simulink model "HANcoder_E407_TTA_Controller_v3"  (R2018b)
settings: Solver=FixedStepDiscrete  StartTime=0.0  StopTime=1  FixedStep=0.01  RelTol=1e-3
PreLoadFcn:
  | librarySetup
  | eval([bdroot,'_startup']) %Calling [modelName]_startup.m
values from neighbouring files (symbols this model uses):
  basic_cycle_duration_bc0 = TM_Reset_Board   + COMP_duration    (= 212)    [HANcoder_E407_TTA_Controller_v3_5_startup.m]    (also in HANcoder_E407_TTA_Controller_v4_6_startup.m; HANcoder_E407_TTA_Controller_v4_7_startup.m; HANcoder_E407_TTA_Controller_v4_startup.m)
  basic_cycle_duration_bc1 = TM_Reset_Var_bc1 + COMP_duration    (= 288)    [HANcoder_E407_TTA_Controller_v3_5_startup.m]    (also in HANcoder_E407_TTA_Controller_v4_6_startup.m = 332; HANcoder_E407_TTA_Controller_v4_7_startup.m = 372; HANcoder_E407_TTA_Controller_v4_startup.m = 332)
  comm_delay_estimation1 = round(comm_delay_measured1*hardware_granularity/frequency_IRQ)    [HANcoder_E407_TTA_Controller_v3_5_startup.m]    (also in HANcoder_E407_TTA_Controller_v4_6_startup.m; HANcoder_E407_TTA_Controller_v4_7_startup.m; HANcoder_E407_TTA_Controller_v4_startup.m)
  comm_delay_estimation2 = round(comm_delay_measured2*hardware_granularity/frequency_IRQ)    [HANcoder_E407_TTA_Controller_v3_5_startup.m]    (also in HANcoder_E407_TTA_Controller_v4_6_startup.m; HANcoder_E407_TTA_Controller_v4_7_startup.m; HANcoder_E407_TTA_Controller_v4_startup.m)
  COMM_Period = 40    [HANcoder_E407_TTA_Controller_v3_5_startup.m]    (also in HANcoder_E407_TTA_Controller_v4_6_startup.m; HANcoder_E407_TTA_Controller_v4_7_startup.m; HANcoder_E407_TTA_Controller_v4_startup.m)
  COMM_Phase1 = Simulink.Parameter    [HANcoder_E407_TTA_Controller_v3_5_startup.m]    (also in HANcoder_E407_TTA_Controller_v4_6_startup.m; HANcoder_E407_TTA_Controller_v4_7_startup.m; HANcoder_E407_TTA_Controller_v4_startup.m)
  COMM_Phase2 = Simulink.Parameter    [HANcoder_E407_TTA_Controller_v3_5_startup.m]    (also in HANcoder_E407_TTA_Controller_v4_6_startup.m; HANcoder_E407_TTA_Controller_v4_7_startup.m; HANcoder_E407_TTA_Controller_v4_startup.m)
  COMM_Phase_init1 = Simulink.Parameter    [HANcoder_E407_TTA_Controller_v3_5_startup.m]    (also in HANcoder_E407_TTA_Controller_v4_6_startup.m; HANcoder_E407_TTA_Controller_v4_7_startup.m; HANcoder_E407_TTA_Controller_v4_startup.m)
  COMM_Phase_init2 = Simulink.Parameter    [HANcoder_E407_TTA_Controller_v3_5_startup.m]    (also in HANcoder_E407_TTA_Controller_v4_6_startup.m; HANcoder_E407_TTA_Controller_v4_7_startup.m; HANcoder_E407_TTA_Controller_v4_startup.m)
  COMP_duration = 4    [HANcoder_E407_TTA_Controller_v3_5_startup.m]    (also in HANcoder_E407_TTA_Controller_v4_6_startup.m; HANcoder_E407_TTA_Controller_v4_7_startup.m; HANcoder_E407_TTA_Controller_v4_startup.m)
  Controller1_Board = 1    [HANcoder_E407_TTA_Controller_v3_5_startup.m]    (also in HANcoder_E407_TTA_Controller_v4_6_startup.m; HANcoder_E407_TTA_Controller_v4_7_startup.m; HANcoder_E407_TTA_Controller_v4_startup.m)
  Controller2_Board = 2    [HANcoder_E407_TTA_Controller_v3_5_startup.m]    (also in HANcoder_E407_TTA_Controller_v4_6_startup.m; HANcoder_E407_TTA_Controller_v4_7_startup.m; HANcoder_E407_TTA_Controller_v4_startup.m)
  Controller3_Board = 3    [HANcoder_E407_TTA_Controller_v3_5_startup.m]    (also in HANcoder_E407_TTA_Controller_v4_6_startup.m; HANcoder_E407_TTA_Controller_v4_7_startup.m; HANcoder_E407_TTA_Controller_v4_startup.m)
  delta_a_set = Simulink.Parameter    [HANcoder_E407_TTA_Controller_v3_5_startup.m]    (also in HANcoder_E407_TTA_Controller_v4_6_startup.m; HANcoder_E407_TTA_Controller_v4_7_startup.m; HANcoder_E407_TTA_Controller_v4_startup.m)
  delta_f_set = Simulink.Parameter    [HANcoder_E407_TTA_Controller_v3_5_startup.m]    (also in HANcoder_E407_TTA_Controller_v4_6_startup.m; HANcoder_E407_TTA_Controller_v4_7_startup.m; HANcoder_E407_TTA_Controller_v4_startup.m)
  delta_max = 1    [HANcoder_E407_TTA_Controller_v3_5_startup.m]    (also in HANcoder_E407_TTA_Controller_v4_6_startup.m; HANcoder_E407_TTA_Controller_v4_7_startup.m; HANcoder_E407_TTA_Controller_v4_startup.m)
  delta_min = -1    [HANcoder_E407_TTA_Controller_v3_5_startup.m]    (also in HANcoder_E407_TTA_Controller_v4_6_startup.m; HANcoder_E407_TTA_Controller_v4_7_startup.m; HANcoder_E407_TTA_Controller_v4_startup.m)
  delta_precision = 6    [HANcoder_E407_TTA_Controller_v3_5_startup.m]    (also in HANcoder_E407_TTA_Controller_v4_6_startup.m; HANcoder_E407_TTA_Controller_v4_7_startup.m; HANcoder_E407_TTA_Controller_v4_startup.m)
  e_width = 0.1    [HANcoder_E407_TTA_Controller_v3_5_startup.m]    (also in HANcoder_E407_TTA_Controller_v4_6_startup.m; HANcoder_E407_TTA_Controller_v4_7_startup.m; HANcoder_E407_TTA_Controller_v4_startup.m)
  frequency_IRQ = 100    [HANcoder_E407_2xCAN_TEST_startup.m]    (also in HANcoder_E407_TTA_Controller_v3_5_startup.m; HANcoder_E407_TTA_Controller_v4_6_startup.m; HANcoder_E407_TTA_Controller_v4_7_startup.m; HANcoder_E407_TTA_Controller_v4_startup.m)
  HANtuneOverride = Simulink.Parameter    [HANcoder_E407_2xCAN_TEST_startup.m]    (also in HANcoder_E407_TTA_Controller_v3_5_startup.m; HANcoder_E407_TTA_Controller_v4_6_startup.m; HANcoder_E407_TTA_Controller_v4_7_startup.m; HANcoder_E407_TTA_Controller_v4_startup.m)
  hardware_granularity = 1000000    [HANcoder_E407_2xCAN_TEST_startup.m]    (also in HANcoder_E407_TTA_Controller_v3_5_startup.m; HANcoder_E407_TTA_Controller_v4_6_startup.m; HANcoder_E407_TTA_Controller_v4_7_startup.m; HANcoder_E407_TTA_Controller_v4_startup.m)
  I_a = 2.25    [HANcoder_E407_TTA_Controller_v3_5_startup.m]    (also in HANcoder_E407_TTA_Controller_v4_6_startup.m; HANcoder_E407_TTA_Controller_v4_7_startup.m; HANcoder_E407_TTA_Controller_v4_startup.m)
  I_f = 2.25    [HANcoder_E407_TTA_Controller_v3_5_startup.m]    (also in HANcoder_E407_TTA_Controller_v4_6_startup.m; HANcoder_E407_TTA_Controller_v4_7_startup.m; HANcoder_E407_TTA_Controller_v4_startup.m)
  idle_time_init = basic_cycle_duration_bc0 + basic_cycle_duration_bc1    (= 500)    [HANcoder_E407_TTA_Controller_v3_5_startup.m]    (also in HANcoder_E407_TTA_Controller_v4_6_startup.m = 544; HANcoder_E407_TTA_Controller_v4_7_startup.m = 584; HANcoder_E407_TTA_Controller_v4_startup.m = 544)
  Input_Gen_Board = 4    [HANcoder_E407_TTA_Controller_v3_5_startup.m]    (also in HANcoder_E407_TTA_Controller_v4_6_startup.m; HANcoder_E407_TTA_Controller_v4_7_startup.m; HANcoder_E407_TTA_Controller_v4_startup.m)
  LA_Clock_Gr = 1    [HANcoder_E407_TTA_Controller_v3_5_startup.m]    (also in HANcoder_E407_TTA_Controller_v4_6_startup.m; HANcoder_E407_TTA_Controller_v4_7_startup.m; HANcoder_E407_TTA_Controller_v4_startup.m)
  LA_COMM_dly = 1    [HANcoder_E407_TTA_Controller_v3_5_startup.m]    (also in HANcoder_E407_TTA_Controller_v4_6_startup.m; HANcoder_E407_TTA_Controller_v4_7_startup.m; HANcoder_E407_TTA_Controller_v4_startup.m)
  LA_COMM_Err = 1    [HANcoder_E407_TTA_Controller_v3_5_startup.m]    (also in HANcoder_E407_TTA_Controller_v4_6_startup.m; HANcoder_E407_TTA_Controller_v4_7_startup.m; HANcoder_E407_TTA_Controller_v4_startup.m)
  LA_E_Desync = 1    [HANcoder_E407_TTA_Controller_v3_5_startup.m]    (also in HANcoder_E407_TTA_Controller_v4_6_startup.m; HANcoder_E407_TTA_Controller_v4_7_startup.m; HANcoder_E407_TTA_Controller_v4_startup.m)
  LA_MEX_Flag = 1    [HANcoder_E407_TTA_Controller_v3_5_startup.m]    (also in HANcoder_E407_TTA_Controller_v4_6_startup.m; HANcoder_E407_TTA_Controller_v4_7_startup.m; HANcoder_E407_TTA_Controller_v4_startup.m)
  LA_Task_Act = 1    [HANcoder_E407_TTA_Controller_v3_5_startup.m]    (also in HANcoder_E407_TTA_Controller_v4_6_startup.m; HANcoder_E407_TTA_Controller_v4_7_startup.m; HANcoder_E407_TTA_Controller_v4_startup.m)
  m_v = 100.0    (= 100)    [HANcoder_E407_TTA_Controller_v3_5_startup.m]    (also in HANcoder_E407_TTA_Controller_v4_6_startup.m; HANcoder_E407_TTA_Controller_v4_7_startup.m; HANcoder_E407_TTA_Controller_v4_startup.m)
  Master_Role = 1    [HANcoder_E407_TTA_Controller_v3_5_startup.m]    (also in HANcoder_E407_TTA_Controller_v4_6_startup.m; HANcoder_E407_TTA_Controller_v4_7_startup.m; HANcoder_E407_TTA_Controller_v4_startup.m)
  matrix_cycle_duration = basic_cycle_duration_bc0 + basic_cycle_duration_bc1    (= 500)    [HANcoder_E407_TTA_Controller_v3_5_startup.m]    (also in HANcoder_E407_TTA_Controller_v4_6_startup.m = 544; HANcoder_E407_TTA_Controller_v4_7_startup.m = 584; HANcoder_E407_TTA_Controller_v4_startup.m = 544)
  matrix_rows = 2    [HANcoder_E407_TTA_Controller_v3_5_startup.m]    (also in HANcoder_E407_TTA_Controller_v4_6_startup.m; HANcoder_E407_TTA_Controller_v4_7_startup.m; HANcoder_E407_TTA_Controller_v4_startup.m)
  max_desync = 15    [HANcoder_E407_TTA_Controller_v3_5_startup.m]    (also in HANcoder_E407_TTA_Controller_v4_6_startup.m; HANcoder_E407_TTA_Controller_v4_7_startup.m = 30; HANcoder_E407_TTA_Controller_v4_startup.m)
  max_num_msgs_CAN1 = 2^Tx_bit_number-1    (= 7)    [HANcoder_E407_TTA_Controller_v3_5_startup.m]    (also in HANcoder_E407_TTA_Controller_v4_6_startup.m = 15; HANcoder_E407_TTA_Controller_v4_7_startup.m = 15; HANcoder_E407_TTA_Controller_v4_startup.m)
  max_num_msgs_CAN2 = max_num_msgs_CAN1    (= 7)    [HANcoder_E407_TTA_Controller_v3_5_startup.m]    (also in HANcoder_E407_TTA_Controller_v4_6_startup.m = 15; HANcoder_E407_TTA_Controller_v4_7_startup.m = 15; HANcoder_E407_TTA_Controller_v4_startup.m)
  min_desync = (-1)*max_desync    (= -15)    [HANcoder_E407_TTA_Controller_v3_5_startup.m]    (also in HANcoder_E407_TTA_Controller_v4_6_startup.m; HANcoder_E407_TTA_Controller_v4_7_startup.m = -30; HANcoder_E407_TTA_Controller_v4_startup.m)
  OutControl1_ID = 23    [HANcoder_E407_TTA_Controller_v3_5_startup.m]    (also in HANcoder_E407_TTA_Controller_v4_6_startup.m; HANcoder_E407_TTA_Controller_v4_7_startup.m; HANcoder_E407_TTA_Controller_v4_startup.m)
  OutControl2_ID = 24    [HANcoder_E407_TTA_Controller_v3_5_startup.m]    (also in HANcoder_E407_TTA_Controller_v4_6_startup.m; HANcoder_E407_TTA_Controller_v4_7_startup.m; HANcoder_E407_TTA_Controller_v4_startup.m)
  OutEmulator_ID = 25    [HANcoder_E407_TTA_Controller_v3_5_startup.m]    (also in HANcoder_E407_TTA_Controller_v4_6_startup.m = 26; HANcoder_E407_TTA_Controller_v4_7_startup.m = 26; HANcoder_E407_TTA_Controller_v4_startup.m)
  R_al = 0.10    (= 0.1)    [HANcoder_E407_TTA_Controller_v3_5_startup.m]    (also in HANcoder_E407_TTA_Controller_v4_6_startup.m; HANcoder_E407_TTA_Controller_v4_7_startup.m; HANcoder_E407_TTA_Controller_v4_startup.m)
  R_ar = 0.10    (= 0.1)    [HANcoder_E407_TTA_Controller_v3_5_startup.m]    (also in HANcoder_E407_TTA_Controller_v4_6_startup.m; HANcoder_E407_TTA_Controller_v4_7_startup.m; HANcoder_E407_TTA_Controller_v4_startup.m)
  R_fl = 0.10    (= 0.1)    [HANcoder_E407_TTA_Controller_v3_5_startup.m]    (also in HANcoder_E407_TTA_Controller_v4_6_startup.m; HANcoder_E407_TTA_Controller_v4_7_startup.m; HANcoder_E407_TTA_Controller_v4_startup.m)
  R_fr = 0.10    (= 0.1)    [HANcoder_E407_TTA_Controller_v3_5_startup.m]    (also in HANcoder_E407_TTA_Controller_v4_6_startup.m; HANcoder_E407_TTA_Controller_v4_7_startup.m; HANcoder_E407_TTA_Controller_v4_startup.m)
  script_run = Simulink.Parameter    [HANcoder_E407_TTA_Controller_v3_5_startup.m]    (also in HANcoder_E407_TTA_Controller_v4_6_startup.m; HANcoder_E407_TTA_Controller_v4_7_startup.m; HANcoder_E407_TTA_Controller_v4_startup.m)
  SensorValues_ID = 22    [HANcoder_E407_TTA_Controller_v3_5_startup.m]    (also in HANcoder_E407_TTA_Controller_v4_6_startup.m; HANcoder_E407_TTA_Controller_v4_7_startup.m; HANcoder_E407_TTA_Controller_v4_startup.m)
  SetValues_ID = 21    [HANcoder_E407_TTA_Controller_v3_5_startup.m]    (also in HANcoder_E407_TTA_Controller_v4_6_startup.m; HANcoder_E407_TTA_Controller_v4_7_startup.m; HANcoder_E407_TTA_Controller_v4_startup.m)
  Slave_Role = 2    [HANcoder_E407_TTA_Controller_v3_5_startup.m]    (also in HANcoder_E407_TTA_Controller_v4_6_startup.m; HANcoder_E407_TTA_Controller_v4_7_startup.m; HANcoder_E407_TTA_Controller_v4_startup.m)
  speed_k_d = Simulink.Parameter    [HANcoder_E407_TTA_Controller_v3_5_startup.m]    (also in HANcoder_E407_TTA_Controller_v4_6_startup.m; HANcoder_E407_TTA_Controller_v4_7_startup.m; HANcoder_E407_TTA_Controller_v4_startup.m)
  speed_k_i = Simulink.Parameter    [HANcoder_E407_TTA_Controller_v3_5_startup.m]    (also in HANcoder_E407_TTA_Controller_v4_6_startup.m; HANcoder_E407_TTA_Controller_v4_7_startup.m; HANcoder_E407_TTA_Controller_v4_startup.m)
  speed_k_p = Simulink.Parameter    [HANcoder_E407_TTA_Controller_v3_5_startup.m]    (also in HANcoder_E407_TTA_Controller_v4_6_startup.m; HANcoder_E407_TTA_Controller_v4_7_startup.m; HANcoder_E407_TTA_Controller_v4_startup.m)
  speed_max = 10    [HANcoder_E407_TTA_Controller_v3_5_startup.m]    (also in HANcoder_E407_TTA_Controller_v4_6_startup.m; HANcoder_E407_TTA_Controller_v4_7_startup.m; HANcoder_E407_TTA_Controller_v4_startup.m)
  speed_min = -10    [HANcoder_E407_TTA_Controller_v3_5_startup.m]    (also in HANcoder_E407_TTA_Controller_v4_6_startup.m; HANcoder_E407_TTA_Controller_v4_7_startup.m; HANcoder_E407_TTA_Controller_v4_startup.m)
  speed_precision = 3    [HANcoder_E407_TTA_Controller_v3_5_startup.m]    (also in HANcoder_E407_TTA_Controller_v4_6_startup.m; HANcoder_E407_TTA_Controller_v4_7_startup.m; HANcoder_E407_TTA_Controller_v4_startup.m)
  Sync_ID = 1    [HANcoder_E407_TTA_Controller_v3_5_startup.m]    (also in HANcoder_E407_TTA_Controller_v4_6_startup.m; HANcoder_E407_TTA_Controller_v4_7_startup.m; HANcoder_E407_TTA_Controller_v4_startup.m)
  tau_max = 5    [HANcoder_E407_TTA_Controller_v3_5_startup.m]    (also in HANcoder_E407_TTA_Controller_v4_6_startup.m; HANcoder_E407_TTA_Controller_v4_7_startup.m; HANcoder_E407_TTA_Controller_v4_startup.m)
  tau_min = -5    [HANcoder_E407_TTA_Controller_v3_5_startup.m]    (also in HANcoder_E407_TTA_Controller_v4_6_startup.m; HANcoder_E407_TTA_Controller_v4_7_startup.m; HANcoder_E407_TTA_Controller_v4_startup.m)
  tau_range = abs(tau_max) + abs(tau_min)    [HANcoder_E407_TTA_Controller_v3_5_startup.m]    (also in HANcoder_E407_TTA_Controller_v4_6_startup.m; HANcoder_E407_TTA_Controller_v4_7_startup.m; HANcoder_E407_TTA_Controller_v4_startup.m)
  theta_max = (speed_max/R_fr)*matrix_cycle_duration*frequency_IRQ/hardware_granularity    (= 5)    [HANcoder_E407_TTA_Controller_v3_5_startup.m]    (also in HANcoder_E407_TTA_Controller_v4_6_startup.m = 5.44; HANcoder_E407_TTA_Controller_v4_7_startup.m = 5.84; HANcoder_E407_TTA_Controller_v4_startup.m = 5.44)
  theta_min = (-1)*theta_max    (= -5)    [HANcoder_E407_TTA_Controller_v3_5_startup.m]    (also in HANcoder_E407_TTA_Controller_v4_6_startup.m = -5.44; HANcoder_E407_TTA_Controller_v4_7_startup.m = -5.84; HANcoder_E407_TTA_Controller_v4_startup.m = -5.44)
  theta_precision = 7-(fix(log2(theta_max))+1)    [HANcoder_E407_TTA_Controller_v3_5_startup.m]    (also in HANcoder_E407_TTA_Controller_v4_6_startup.m; HANcoder_E407_TTA_Controller_v4_7_startup.m; HANcoder_E407_TTA_Controller_v4_startup.m)
  Tl_a = 0.6    [HANcoder_E407_TTA_Controller_v3_5_startup.m]    (also in HANcoder_E407_TTA_Controller_v4_6_startup.m; HANcoder_E407_TTA_Controller_v4_7_startup.m; HANcoder_E407_TTA_Controller_v4_startup.m)
  Tl_f = 0.6    [HANcoder_E407_TTA_Controller_v3_5_startup.m]    (also in HANcoder_E407_TTA_Controller_v4_6_startup.m; HANcoder_E407_TTA_Controller_v4_7_startup.m; HANcoder_E407_TTA_Controller_v4_startup.m)
  TM_Check_Output_Control1 = TM_COMM_Output_Control1 + COMM_duration    (= 188)    [HANcoder_E407_TTA_Controller_v3_5_startup.m]    (also in HANcoder_E407_TTA_Controller_v4_6_startup.m; HANcoder_E407_TTA_Controller_v4_7_startup.m; HANcoder_E407_TTA_Controller_v4_startup.m)
  TM_Check_Output_Control2 = TM_COMM_Output_Control2 + COMM_duration    (= 232)    [HANcoder_E407_TTA_Controller_v3_5_startup.m]    (also in HANcoder_E407_TTA_Controller_v4_6_startup.m; HANcoder_E407_TTA_Controller_v4_7_startup.m; HANcoder_E407_TTA_Controller_v4_startup.m)
  TM_Check_Output_Emulator = TM_COMM_Output_Emulator + COMM_duration    (= 280)    [HANcoder_E407_TTA_Controller_v3_5_startup.m]    (also in HANcoder_E407_TTA_Controller_v4_6_startup.m = 320; HANcoder_E407_TTA_Controller_v4_7_startup.m = 360; HANcoder_E407_TTA_Controller_v4_startup.m = 320)
  TM_Check_Output_Emulator_2 = TM_Check_Output_Emulator + 2    (= 282)    [HANcoder_E407_TTA_Controller_v3_5_startup.m]    (also in HANcoder_E407_TTA_Controller_v4_6_startup.m = 322; HANcoder_E407_TTA_Controller_v4_7_startup.m = 362; HANcoder_E407_TTA_Controller_v4_startup.m = 322)
  TM_Check_Sensor_Values = TM_COMM_Sensor_Values + COMM_duration    (= 132)    [HANcoder_E407_TTA_Controller_v3_5_startup.m]    (also in HANcoder_E407_TTA_Controller_v4_6_startup.m; HANcoder_E407_TTA_Controller_v4_7_startup.m; HANcoder_E407_TTA_Controller_v4_startup.m)
  TM_Check_Sensor_Values_2 = TM_Check_Sensor_Values + 2    (= 134)    [HANcoder_E407_TTA_Controller_v3_5_startup.m]    (also in HANcoder_E407_TTA_Controller_v4_6_startup.m; HANcoder_E407_TTA_Controller_v4_7_startup.m; HANcoder_E407_TTA_Controller_v4_startup.m)
  TM_Check_Set_Values = TM_COMM_Set_Values + COMM_duration    (= 88)    [HANcoder_E407_TTA_Controller_v3_5_startup.m]    (also in HANcoder_E407_TTA_Controller_v4_6_startup.m; HANcoder_E407_TTA_Controller_v4_7_startup.m; HANcoder_E407_TTA_Controller_v4_startup.m)
  TM_Check_Set_Values_2 = TM_Check_Set_Values + 2    (= 90)    [HANcoder_E407_TTA_Controller_v3_5_startup.m]    (also in HANcoder_E407_TTA_Controller_v4_6_startup.m; HANcoder_E407_TTA_Controller_v4_7_startup.m; HANcoder_E407_TTA_Controller_v4_startup.m)
  TM_Check_Sync = TM_COMM_Sync   + COMM_duration    (= 40)    [HANcoder_E407_TTA_Controller_v3_5_startup.m]    (also in HANcoder_E407_TTA_Controller_v4_6_startup.m; HANcoder_E407_TTA_Controller_v4_7_startup.m; HANcoder_E407_TTA_Controller_v4_startup.m)
  TM_Check_TOuts = TM_Count_Vote3 + COMP_duration    (= 196)    [HANcoder_E407_TTA_Controller_v3_5_startup.m]    (also in HANcoder_E407_TTA_Controller_v4_6_startup.m; HANcoder_E407_TTA_Controller_v4_7_startup.m; HANcoder_E407_TTA_Controller_v4_startup.m)
  TM_Check_Vote1 = TM_COMM_Vote1  + COMM_duration    (= 92)    [HANcoder_E407_TTA_Controller_v3_5_startup.m]    (also in HANcoder_E407_TTA_Controller_v4_6_startup.m; HANcoder_E407_TTA_Controller_v4_7_startup.m; HANcoder_E407_TTA_Controller_v4_startup.m)
  TM_Check_Vote2 = TM_COMM_Vote2  + COMM_duration    (= 140)    [HANcoder_E407_TTA_Controller_v3_5_startup.m]    (also in HANcoder_E407_TTA_Controller_v4_6_startup.m; HANcoder_E407_TTA_Controller_v4_7_startup.m; HANcoder_E407_TTA_Controller_v4_startup.m)
  TM_Check_Vote2_2 = TM_Check_Vote2 + 2    (= 142)    [HANcoder_E407_TTA_Controller_v3_5_startup.m]    (also in HANcoder_E407_TTA_Controller_v4_6_startup.m; HANcoder_E407_TTA_Controller_v4_7_startup.m; HANcoder_E407_TTA_Controller_v4_startup.m)
  TM_Check_Vote3 = TM_COMM_Vote3  + COMM_duration    (= 188)    [HANcoder_E407_TTA_Controller_v3_5_startup.m]    (also in HANcoder_E407_TTA_Controller_v4_6_startup.m; HANcoder_E407_TTA_Controller_v4_7_startup.m; HANcoder_E407_TTA_Controller_v4_startup.m)
  TM_COMM_Output_Control1 = TM_Velocity + COMP_duration    (= 148)    [HANcoder_E407_TTA_Controller_v3_5_startup.m]    (also in HANcoder_E407_TTA_Controller_v4_6_startup.m; HANcoder_E407_TTA_Controller_v4_7_startup.m; HANcoder_E407_TTA_Controller_v4_startup.m)
  TM_COMM_Output_Control2 = TM_Check_Output_Control1 + COMP_duration    (= 192)    [HANcoder_E407_TTA_Controller_v3_5_startup.m]    (also in HANcoder_E407_TTA_Controller_v4_6_startup.m; HANcoder_E407_TTA_Controller_v4_7_startup.m; HANcoder_E407_TTA_Controller_v4_startup.m)
  TM_COMM_Output_Emulator = TM_TMR + COMP_duration    (= 240)    [HANcoder_E407_TTA_Controller_v3_5_startup.m]    (also in HANcoder_E407_TTA_Controller_v4_6_startup.m = 280; HANcoder_E407_TTA_Controller_v4_7_startup.m = 320; HANcoder_E407_TTA_Controller_v4_startup.m = 280)
  TM_COMM_Sensor_Values = TM_Check_Set_Values + COMP_duration    (= 92)    [HANcoder_E407_TTA_Controller_v3_5_startup.m]    (also in HANcoder_E407_TTA_Controller_v4_6_startup.m; HANcoder_E407_TTA_Controller_v4_7_startup.m; HANcoder_E407_TTA_Controller_v4_startup.m)
  TM_COMM_Set_Values = TM_Update_LT + COMP_duration    (= 48)    [HANcoder_E407_TTA_Controller_v3_5_startup.m]    (also in HANcoder_E407_TTA_Controller_v4_6_startup.m; HANcoder_E407_TTA_Controller_v4_7_startup.m; HANcoder_E407_TTA_Controller_v4_startup.m)
  TM_COMM_Sync = basic_cycle_start    (= 0)    [HANcoder_E407_TTA_Controller_v3_5_startup.m]    (also in HANcoder_E407_TTA_Controller_v4_6_startup.m; HANcoder_E407_TTA_Controller_v4_7_startup.m; HANcoder_E407_TTA_Controller_v4_startup.m)
  TM_COMM_Vote1 = TM_Vote_Dec    + COMP_duration    (= 52)    [HANcoder_E407_TTA_Controller_v3_5_startup.m]    (also in HANcoder_E407_TTA_Controller_v4_6_startup.m; HANcoder_E407_TTA_Controller_v4_7_startup.m; HANcoder_E407_TTA_Controller_v4_startup.m)
  TM_COMM_Vote2 = TM_Count_Vote1 + COMP_duration    (= 100)    [HANcoder_E407_TTA_Controller_v3_5_startup.m]    (also in HANcoder_E407_TTA_Controller_v4_6_startup.m; HANcoder_E407_TTA_Controller_v4_7_startup.m; HANcoder_E407_TTA_Controller_v4_startup.m)
  TM_COMM_Vote3 = TM_Count_Vote2 + COMP_duration    (= 148)    [HANcoder_E407_TTA_Controller_v3_5_startup.m]    (also in HANcoder_E407_TTA_Controller_v4_6_startup.m; HANcoder_E407_TTA_Controller_v4_7_startup.m; HANcoder_E407_TTA_Controller_v4_startup.m)
  TM_Count_Vote1 = TM_Check_Vote1 + COMP_duration    (= 96)    [HANcoder_E407_TTA_Controller_v3_5_startup.m]    (also in HANcoder_E407_TTA_Controller_v4_6_startup.m; HANcoder_E407_TTA_Controller_v4_7_startup.m; HANcoder_E407_TTA_Controller_v4_startup.m)
  TM_Count_Vote2 = TM_Check_Vote2 + COMP_duration    (= 144)    [HANcoder_E407_TTA_Controller_v3_5_startup.m]    (also in HANcoder_E407_TTA_Controller_v4_6_startup.m; HANcoder_E407_TTA_Controller_v4_7_startup.m; HANcoder_E407_TTA_Controller_v4_startup.m)
  TM_Count_Vote3 = TM_Check_Vote3 + COMP_duration    (= 192)    [HANcoder_E407_TTA_Controller_v3_5_startup.m]    (also in HANcoder_E407_TTA_Controller_v4_6_startup.m; HANcoder_E407_TTA_Controller_v4_7_startup.m; HANcoder_E407_TTA_Controller_v4_startup.m)
  TM_Data_bc0 = TM_COMM_Sync    (= 0)    [HANcoder_E407_TTA_Controller_v3_5_startup.m]    (also in HANcoder_E407_TTA_Controller_v4_6_startup.m; HANcoder_E407_TTA_Controller_v4_7_startup.m; HANcoder_E407_TTA_Controller_v4_startup.m)
  TM_Data_bc1 = TM_Data_bc0(1:4)    [HANcoder_E407_TTA_Controller_v3_5_startup.m]    (also in HANcoder_E407_TTA_Controller_v4_6_startup.m; HANcoder_E407_TTA_Controller_v4_7_startup.m; HANcoder_E407_TTA_Controller_v4_startup.m)
  TM_New_Master = TM_Check_TOuts + COMP_duration    (= 200)    [HANcoder_E407_TTA_Controller_v3_5_startup.m]    (also in HANcoder_E407_TTA_Controller_v4_6_startup.m; HANcoder_E407_TTA_Controller_v4_7_startup.m; HANcoder_E407_TTA_Controller_v4_startup.m)
  TM_Reset_Board = TM_Reset_Var   + COMP_duration    (= 208)    [HANcoder_E407_TTA_Controller_v3_5_startup.m]    (also in HANcoder_E407_TTA_Controller_v4_6_startup.m; HANcoder_E407_TTA_Controller_v4_7_startup.m; HANcoder_E407_TTA_Controller_v4_startup.m)
  TM_Reset_Var = TM_New_Master  + COMP_duration    (= 204)    [HANcoder_E407_TTA_Controller_v3_5_startup.m]    (also in HANcoder_E407_TTA_Controller_v4_6_startup.m; HANcoder_E407_TTA_Controller_v4_7_startup.m; HANcoder_E407_TTA_Controller_v4_startup.m)
  TM_Reset_Var_bc1 = TM_Check_Output_Emulator + COMP_duration    (= 284)    [HANcoder_E407_TTA_Controller_v3_5_startup.m]    (also in HANcoder_E407_TTA_Controller_v4_6_startup.m = 328; HANcoder_E407_TTA_Controller_v4_7_startup.m = 368; HANcoder_E407_TTA_Controller_v4_startup.m = 328)
  TM_Reset_Var_bc1_2 = TM_Reset_Var_bc1 + 2    (= 286)    [HANcoder_E407_TTA_Controller_v3_5_startup.m]    (also in HANcoder_E407_TTA_Controller_v4_6_startup.m = 330; HANcoder_E407_TTA_Controller_v4_7_startup.m = 370; HANcoder_E407_TTA_Controller_v4_startup.m = 330)
  TM_Steer = TM_Check_Sensor_Values + COMP_duration    (= 136)    [HANcoder_E407_TTA_Controller_v3_5_startup.m]    (also in HANcoder_E407_TTA_Controller_v4_6_startup.m; HANcoder_E407_TTA_Controller_v4_7_startup.m; HANcoder_E407_TTA_Controller_v4_startup.m)
  TM_TMR = TM_Check_Output_Control2 + COMP_duration    (= 236)    [HANcoder_E407_TTA_Controller_v3_5_startup.m]    (also in HANcoder_E407_TTA_Controller_v4_6_startup.m = 276; HANcoder_E407_TTA_Controller_v4_7_startup.m = 316; HANcoder_E407_TTA_Controller_v4_startup.m = 276)
  TM_TMR_2 = TM_TMR + 1    (= 237)    [HANcoder_E407_TTA_Controller_v3_5_startup.m]    (also in HANcoder_E407_TTA_Controller_v4_6_startup.m = 277; HANcoder_E407_TTA_Controller_v4_7_startup.m = 317; HANcoder_E407_TTA_Controller_v4_startup.m = 277)
  TM_TMR_3 = TM_TMR + 3    (= 239)    [HANcoder_E407_TTA_Controller_v3_5_startup.m]    (also in HANcoder_E407_TTA_Controller_v4_6_startup.m = 279; HANcoder_E407_TTA_Controller_v4_7_startup.m = 319; HANcoder_E407_TTA_Controller_v4_startup.m = 279)
  TM_Torque = TM_Steer + COMP_duration    (= 140)    [HANcoder_E407_TTA_Controller_v3_5_startup.m]    (also in HANcoder_E407_TTA_Controller_v4_6_startup.m; HANcoder_E407_TTA_Controller_v4_7_startup.m; HANcoder_E407_TTA_Controller_v4_startup.m)
  TM_Type_bc0 = COMM    (= 0)    [HANcoder_E407_TTA_Controller_v3_5_startup.m]    (also in HANcoder_E407_TTA_Controller_v4_6_startup.m; HANcoder_E407_TTA_Controller_v4_7_startup.m; HANcoder_E407_TTA_Controller_v4_startup.m)
  TM_Type_bc1 = TM_Type_bc0(1:4)    [HANcoder_E407_TTA_Controller_v3_5_startup.m]    (also in HANcoder_E407_TTA_Controller_v4_6_startup.m; HANcoder_E407_TTA_Controller_v4_7_startup.m; HANcoder_E407_TTA_Controller_v4_startup.m)
  TM_Update_LT = TM_Check_Sync  + COMP_duration    (= 44)    [HANcoder_E407_TTA_Controller_v3_5_startup.m]    (also in HANcoder_E407_TTA_Controller_v4_6_startup.m; HANcoder_E407_TTA_Controller_v4_7_startup.m; HANcoder_E407_TTA_Controller_v4_startup.m)
  TM_Update_LT_2 = TM_Update_LT   + 2    (= 46)    [HANcoder_E407_TTA_Controller_v3_5_startup.m]    (also in HANcoder_E407_TTA_Controller_v4_6_startup.m; HANcoder_E407_TTA_Controller_v4_7_startup.m; HANcoder_E407_TTA_Controller_v4_startup.m)
  TM_Velocity = TM_Torque + COMP_duration    (= 144)    [HANcoder_E407_TTA_Controller_v3_5_startup.m]    (also in HANcoder_E407_TTA_Controller_v4_6_startup.m; HANcoder_E407_TTA_Controller_v4_7_startup.m; HANcoder_E407_TTA_Controller_v4_startup.m)
  TM_Vote_Dec = TM_Update_LT   + COMP_duration    (= 48)    [HANcoder_E407_TTA_Controller_v3_5_startup.m]    (also in HANcoder_E407_TTA_Controller_v4_6_startup.m; HANcoder_E407_TTA_Controller_v4_7_startup.m; HANcoder_E407_TTA_Controller_v4_startup.m)
  TM_Vote_Dec_2 = TM_Vote_Dec    + 2    (= 50)    [HANcoder_E407_TTA_Controller_v3_5_startup.m]    (also in HANcoder_E407_TTA_Controller_v4_6_startup.m; HANcoder_E407_TTA_Controller_v4_7_startup.m; HANcoder_E407_TTA_Controller_v4_startup.m)
  torque_a_k_d = Simulink.Parameter    [HANcoder_E407_TTA_Controller_v3_5_startup.m]    (also in HANcoder_E407_TTA_Controller_v4_6_startup.m; HANcoder_E407_TTA_Controller_v4_7_startup.m; HANcoder_E407_TTA_Controller_v4_startup.m)
  torque_a_k_i = Simulink.Parameter    [HANcoder_E407_TTA_Controller_v3_5_startup.m]    (also in HANcoder_E407_TTA_Controller_v4_6_startup.m; HANcoder_E407_TTA_Controller_v4_7_startup.m; HANcoder_E407_TTA_Controller_v4_startup.m)
  torque_a_k_p = Simulink.Parameter    [HANcoder_E407_TTA_Controller_v3_5_startup.m]    (also in HANcoder_E407_TTA_Controller_v4_6_startup.m; HANcoder_E407_TTA_Controller_v4_7_startup.m; HANcoder_E407_TTA_Controller_v4_startup.m)
  torque_f_k_d = Simulink.Parameter    [HANcoder_E407_TTA_Controller_v3_5_startup.m]    (also in HANcoder_E407_TTA_Controller_v4_6_startup.m; HANcoder_E407_TTA_Controller_v4_7_startup.m; HANcoder_E407_TTA_Controller_v4_startup.m)
  torque_f_k_i = Simulink.Parameter    [HANcoder_E407_TTA_Controller_v3_5_startup.m]    (also in HANcoder_E407_TTA_Controller_v4_6_startup.m; HANcoder_E407_TTA_Controller_v4_7_startup.m; HANcoder_E407_TTA_Controller_v4_startup.m)
  torque_f_k_p = Simulink.Parameter    [HANcoder_E407_TTA_Controller_v3_5_startup.m]    (also in HANcoder_E407_TTA_Controller_v4_6_startup.m; HANcoder_E407_TTA_Controller_v4_7_startup.m; HANcoder_E407_TTA_Controller_v4_startup.m)
  torque_precision = 4    [HANcoder_E407_TTA_Controller_v3_5_startup.m]    (also in HANcoder_E407_TTA_Controller_v4_6_startup.m; HANcoder_E407_TTA_Controller_v4_7_startup.m; HANcoder_E407_TTA_Controller_v4_startup.m)
  v_set = Simulink.Parameter    [HANcoder_E407_TTA_Controller_v3_5_startup.m]    (also in HANcoder_E407_TTA_Controller_v4_6_startup.m; HANcoder_E407_TTA_Controller_v4_7_startup.m; HANcoder_E407_TTA_Controller_v4_startup.m)
  Vehicle_Em_Board = 5    [HANcoder_E407_TTA_Controller_v3_5_startup.m]    (also in HANcoder_E407_TTA_Controller_v4_6_startup.m; HANcoder_E407_TTA_Controller_v4_7_startup.m; HANcoder_E407_TTA_Controller_v4_startup.m)
  ... (+3 more)
undefined symbols (not defined in the file or in its folder): A0, A1, A2, A3, A4, CON2, CON3, CON4, D10, D12, D13, D2, D3, D8, D9
libraries: hdlsllib x352, HANcoder_STM32_Target x30, simulink x3, simulink_extras x1
(part 27 of 65)

== system HANcoder_E407_TTA_Controller_v3/HANcoder STM32 Target - E407-STM32 algorithm/TTA CAN System/TTA System/Matrix Cycle Manager/Controller Matrix Cycle/controller basic cycle 1/COMP Task - Rx_Sensor_Values_Check/Process_Messages ==
  note: Logic Analyzer - DEBUG
      | Sync_Check COMP task
      | activation
  note: Logic Analyzer - DEBUG
  new_CAN1_msg : Inport
  new_CAN2_msg : Inport  Port=2
  Rx_msg_CAN1 : Inport  Port=3  OutDataTypeStr=Bus: msg_buffer_type
  Rx_Msg_CAN2 : Inport  Port=4  OutDataTypeStr=Bus: msg_buffer_type
  expected_board_id : Inport  Port=5
  Enable : EnablePort
  Bus Selector : BusSelector  OutputSignals=signal1,Buffer_2,Buffer_3,Buffer_4,Buffer_5,Buffer_6,Buffer_7,Buffer_8
  Constant2 : Constant  Priority=28  OutDataTypeStr=boolean
  Data Store Write : DataStoreWrite  Priority=4  DataStoreName=Msg_Rx  DataStoreElements=Msg_Rx.Buffer_1#Msg_Rx.Buffer_2#Msg_Rx.Buffer_3#Msg_Rx.Buffer_4#Msg_Rx.Buffer_5#Msg_Rx.Buffer_6#Msg_Rx.Buffer_7#Msg_Rx.Buffer_8
  Data Store Write2 : DataStoreWrite  DataStoreName=new_msg_Rx
  Data Store Write3 : DataStoreWrite  Priority=29  DataStoreName=Toggle_Pin_A0
  Demux message CAN1 and check coherence : Subsystem  Priority=1
  Demux message CAN1 and check coherence1 : Subsystem  Priority=2
  OR : Logic  Operator=OR  IconShape=distinctive  AllPortsSameDT=off  OutDataTypeStr=boolean
  Switch : Switch  Priority=3  Criteria=u2 > Threshold
  Terminator : Terminator
  Terminator1 : Terminator
  wires:
  new_CAN1_msg/1 -> Demux message CAN1 and check coherence/Enable
  new_CAN2_msg/1 -> Demux message CAN1 and check coherence1/Enable
  Rx_msg_CAN1/1 -> Demux message CAN1 and check coherence/1(CAN1_Rx_msg)
  Rx_Msg_CAN2/1 -> Demux message CAN1 and check coherence1/1(CAN2_Rx_msg)
  Demux message CAN1 and check coherence/3(CAN1_msg_coherent) -> Switch/2, OR/1
  Demux message CAN1 and check coherence/1(CAN1_msg) -> Switch/1
  Demux message CAN1 and check coherence1/1(CAN2_msg_coherent) -> OR/2
  Demux message CAN1 and check coherence1/3(CAN2_msg) -> Switch/3
  OR/1 -> Data Store Write2/1
  Constant2/1 -> Data Store Write3/1
  expected_board_id/1 -> Demux message CAN1 and check coherence/2(expected_board_id), Demux message CAN1 and check coherence1/2(expected_board_id)
  Demux message CAN1 and check coherence/2(Msg_Count_CAN1) -> Terminator/1
  Demux message CAN1 and check coherence1/2(Msg_Count_CAN2) -> Terminator1/1
  Bus Selector/5 -> Data Store Write/5  "<Buffer_5>"
  Bus Selector/3 -> Data Store Write/3  "<Buffer_3>"
  Bus Selector/4 -> Data Store Write/4  "<Buffer_4>"
  Bus Selector/7 -> Data Store Write/7  "<Buffer_7>"
  Bus Selector/1 -> Data Store Write/1  "<signal1>"
  Bus Selector/8 -> Data Store Write/8  "<Buffer_8>"
  Bus Selector/6 -> Data Store Write/6  "<Buffer_6>"
  Bus Selector/2 -> Data Store Write/2  "<Buffer_2>"
  Switch/1 -> Bus Selector/1

== system HANcoder_E407_TTA_Controller_v3/HANcoder STM32 Target - E407-STM32 algorithm/TTA CAN System/TTA System/Matrix Cycle Manager/Controller Matrix Cycle/controller basic cycle 1/COMP Task - Rx_Sensor_Values_Check/Reset Tx msg counter ==
  Enable : EnablePort
  Constant1 : Constant  Priority=2
  Constant6 : Constant  Priority=2
  Data Store Write1 : DataStoreWrite  Priority=4  DataStoreName=Tx_msg_count_CAN1
  Data Store Write2 : DataStoreWrite  Priority=4  DataStoreName=Tx_msg_count_CAN2
  wires:
  Constant6/1 -> Data Store Write1/1
  Constant1/1 -> Data Store Write2/1

== system HANcoder_E407_TTA_Controller_v3/HANcoder STM32 Target - E407-STM32 algorithm/TTA CAN System/TTA System/Matrix Cycle Manager/Controller Matrix Cycle/controller basic cycle 1/COMP Task - Rx_Sensor_Values_Check/Update Msg buffer ==
  note: If the msg received is coherent, we update the
      | stored copies of the set values. Otherwise, we
      | do not perform further calculations and raise an error.
  Enable : EnablePort
  Data Store Memory : DataStoreMemory  DataStoreName=mc_counter  ReadBeforeWriteMsg=warning  WriteAfterWriteMsg=warning  WriteAfterReadMsg=warning  InitialValue=1  ShowAdditionalParam=off
  Data Store Read2 : DataStoreRead  DataStoreName=mc_counter
  Data Store Read5 : DataStoreRead  DataStoreName=new_msg_Rx
  Data Store Read6 : DataStoreRead  DataStoreName=Msg_Rx
  NOT1 : Logic  Operator=NOT  IconShape=distinctive  AllPortsSameDT=off  OutDataTypeStr=boolean
  Sensor Values Rx Update : Subsystem  Priority=100  TreatAsAtomicUnit=on
  Sensor Values not Rx Update : Subsystem  Priority=110  TreatAsAtomicUnit=on
  Terminator : Terminator
  wires:
  Data Store Read5/1 -> Sensor Values Rx Update/Enable, NOT1/1  "new_sensor_rx_s"
  Data Store Read6/1 -> Sensor Values Rx Update/1(msg_rx)
  NOT1/1 -> Sensor Values not Rx Update/Enable
  Data Store Read2/1 -> Terminator/1  "mc_counter_s"

== system HANcoder_E407_TTA_Controller_v3/HANcoder STM32 Target - E407-STM32 algorithm/TTA CAN System/TTA System/Matrix Cycle Manager/Controller Matrix Cycle/controller basic cycle 1/COMP Task - Rx_Set_Values_Check/Process_Messages ==
  note: Logic Analyzer - DEBUG
  note: Logic Analyzer - DEBUG
      | Sync_Check COMP task
      | activation
  new_CAN1_msg : Inport
  new_CAN2_msg : Inport  Port=2
  Rx_msg_CAN1 : Inport  Port=3  OutDataTypeStr=Bus: msg_buffer_type
  Rx_Msg_CAN2 : Inport  Port=4  OutDataTypeStr=Bus: msg_buffer_type
  expected_board_id : Inport  Port=5
  Enable : EnablePort
  Bus Selector : BusSelector  OutputSignals=signal1,Buffer_2,Buffer_3,Buffer_4,Buffer_5,Buffer_6,Buffer_7,Buffer_8
  Constant2 : Constant  Priority=28  OutDataTypeStr=boolean
  Data Store Write : DataStoreWrite  Priority=4  DataStoreName=Msg_Rx  DataStoreElements=Msg_Rx.Buffer_1#Msg_Rx.Buffer_2#Msg_Rx.Buffer_3#Msg_Rx.Buffer_4#Msg_Rx.Buffer_5#Msg_Rx.Buffer_6#Msg_Rx.Buffer_7#Msg_Rx.Buffer_8
  Data Store Write1 : DataStoreWrite  DataStoreName=new_msg_Rx
  Data Store Write3 : DataStoreWrite  Priority=29  DataStoreName=Toggle_Pin_A0
  Demux message CAN1 and check coherence : Subsystem  Priority=1
  Demux message CAN1 and check coherence1 : Subsystem  Priority=2
  OR : Logic  Operator=OR  IconShape=distinctive  AllPortsSameDT=off  OutDataTypeStr=boolean
  Switch : Switch  Priority=3  Criteria=u2 > Threshold
  Terminator : Terminator
  Terminator1 : Terminator
  wires:
  Bus Selector/2 -> Data Store Write/2  "<Buffer_2>"
  Bus Selector/6 -> Data Store Write/6  "<Buffer_6>"
  Switch/1 -> Bus Selector/1
  Bus Selector/8 -> Data Store Write/8  "<Buffer_8>"
  Bus Selector/1 -> Data Store Write/1  "<signal1>"
  Bus Selector/7 -> Data Store Write/7  "<Buffer_7>"
  Bus Selector/4 -> Data Store Write/4  "<Buffer_4>"
  Bus Selector/3 -> Data Store Write/3  "<Buffer_3>"
  Bus Selector/5 -> Data Store Write/5  "<Buffer_5>"
  Demux message CAN1 and check coherence1/2(Msg_Count_CAN2) -> Terminator/1
  Demux message CAN1 and check coherence/2(Msg_Count_CAN1) -> Terminator1/1
  expected_board_id/1 -> Demux message CAN1 and check coherence1/2(expected_board_id), Demux message CAN1 and check coherence/2(expected_board_id)
  Constant2/1 -> Data Store Write3/1
  OR/1 -> Data Store Write1/1
  Demux message CAN1 and check coherence1/3(CAN2_msg) -> Switch/3
  Demux message CAN1 and check coherence1/1(CAN2_msg_coherent) -> OR/2
  Demux message CAN1 and check coherence/1(CAN1_msg) -> Switch/1
  Demux message CAN1 and check coherence/3(CAN1_msg_coherent) -> OR/1, Switch/2
  Rx_Msg_CAN2/1 -> Demux message CAN1 and check coherence1/1(CAN2_Rx_msg)
  Rx_msg_CAN1/1 -> Demux message CAN1 and check coherence/1(CAN1_Rx_msg)
  new_CAN2_msg/1 -> Demux message CAN1 and check coherence1/Enable
  new_CAN1_msg/1 -> Demux message CAN1 and check coherence/Enable

== system HANcoder_E407_TTA_Controller_v3/HANcoder STM32 Target - E407-STM32 algorithm/TTA CAN System/TTA System/Matrix Cycle Manager/Controller Matrix Cycle/controller basic cycle 1/COMP Task - Rx_Set_Values_Check/Reset Tx msg counter ==
  Enable : EnablePort
  Constant1 : Constant  Priority=2
  Constant6 : Constant  Priority=2
  Data Store Write1 : DataStoreWrite  Priority=4  DataStoreName=Tx_msg_count_CAN1
  Data Store Write2 : DataStoreWrite  Priority=4  DataStoreName=Tx_msg_count_CAN2
  wires:
  Constant1/1 -> Data Store Write2/1
  Constant6/1 -> Data Store Write1/1

== system HANcoder_E407_TTA_Controller_v3/HANcoder STM32 Target - E407-STM32 algorithm/TTA CAN System/TTA System/Matrix Cycle Manager/Controller Matrix Cycle/controller basic cycle 1/COMP Task - Rx_Set_Values_Check/Update Msg buffer ==
  note: If the msg received is coherent, we update the
      | stored copies of the set values. Otherwise, we
      | do not perform any more calculations and raise an error.
  Enable : EnablePort
  Data Store Read5 : DataStoreRead  DataStoreName=new_msg_Rx
  Data Store Read6 : DataStoreRead  DataStoreName=Msg_Rx
  NOT1 : Logic  Operator=NOT  IconShape=distinctive  AllPortsSameDT=off  OutDataTypeStr=boolean
  Set Values Update : Subsystem  Priority=100  TreatAsAtomicUnit=on
  Set Values not Rx : Subsystem  Priority=100  TreatAsAtomicUnit=on
  wires:
  NOT1/1 -> Set Values not Rx/Enable
  Data Store Read5/1 -> NOT1/1, Set Values Update/Enable  "new_set_rx_s"
  Data Store Read6/1 -> Set Values Update/1(msg_rx)

== system HANcoder_E407_TTA_Controller_v3/HANcoder STM32 Target - E407-STM32 algorithm/TTA CAN System/TTA System/Matrix Cycle Manager/Controller Matrix Cycle/controller basic cycle 1/COMP Task - Sync bc1 check/Process_Messages ==
  note: Logic Analyzer - DEBUG
      | Sync_Check COMP task
      | activation
  note: Logic Analyzer - DEBUG
  new_CAN1_msg : Inport
  new_CAN2_msg : Inport  Port=2
  Rx_msg_CAN1 : Inport  Port=3  OutDataTypeStr=Bus: msg_buffer_type
  Rx_Msg_CAN2 : Inport  Port=4  OutDataTypeStr=Bus: msg_buffer_type
  expected_basic_cycle : Inport  Port=5
  TM_COMM : Inport  Port=6
  expected_board_id : Inport  Port=7
  Enable : EnablePort
  Bus Selector : BusSelector  OutputSignals=signal1,Buffer_2,Buffer_3,Buffer_4,Buffer_5,Buffer_6,Buffer_7,Buffer_8
  Constant2 : Constant  Priority=28  OutDataTypeStr=boolean
  Data Store Write : DataStoreWrite  Priority=4  DataStoreName=Msg_Rx  DataStoreElements=Msg_Rx.Buffer_1#Msg_Rx.Buffer_2#Msg_Rx.Buffer_3#Msg_Rx.Buffer_4#Msg_Rx.Buffer_5#Msg_Rx.Buffer_6#Msg_Rx.Buffer_7#Msg_Rx.Buffer_8
  Data Store Write2 : DataStoreWrite  DataStoreName=new_msg_Rx
  Data Store Write3 : DataStoreWrite  Priority=29  DataStoreName=Toggle_Pin_A0
  Demux message CAN1 and check coherence : Subsystem  Priority=1
  Demux message CAN1 and check coherence1 : Subsystem  Priority=2
  Desync calculation : Subsystem  Priority=10
  OR : Logic  Operator=OR  IconShape=distinctive  AllPortsSameDT=off  OutDataTypeStr=boolean
  Switch : Switch  Priority=3  Criteria=u2 > Threshold
  wires:
  new_CAN1_msg/1 -> Demux message CAN1 and check coherence/Enable
  new_CAN2_msg/1 -> Demux message CAN1 and check coherence1/Enable
  Rx_msg_CAN1/1 -> Demux message CAN1 and check coherence/1(CAN1_Rx_msg)
  Rx_Msg_CAN2/1 -> Demux message CAN1 and check coherence1/1(CAN2_Rx_msg)
  Demux message CAN1 and check coherence/1(CAN1_msg) -> Switch/1
  Demux message CAN1 and check coherence1/1(CAN2_msg_coherent) -> OR/2
  Demux message CAN1 and check coherence1/3(CAN2_msg) -> Switch/3
  expected_basic_cycle/1 -> Demux message CAN1 and check coherence1/2(expected_basic_cycle), Demux message CAN1 and check coherence/2(expected_basic_cycle)
  Constant2/1 -> Data Store Write3/1
  expected_board_id/1 -> Demux message CAN1 and check coherence1/3(expected_board_id), Demux message CAN1 and check coherence/3(expected_board_id)
  Demux message CAN1 and check coherence/2(Msg_Count_CAN1) -> [msg_count_CAN1]
  Demux message CAN1 and check coherence1/2(Msg_Count_CAN2) -> [msg_count_CAN2]
  Switch/1 -> Bus Selector/1
  Bus Selector/1 -> Data Store Write/1  "<signal1>"
  Bus Selector/2 -> Data Store Write/2  "<Buffer_2>"
  Bus Selector/3 -> Data Store Write/3  "<Buffer_3>"
  Bus Selector/4 -> Data Store Write/4  "<Buffer_4>"
  Bus Selector/5 -> Data Store Write/5  "<Buffer_5>"
  Bus Selector/6 -> Data Store Write/6  "<Buffer_6>"
  Bus Selector/7 -> Data Store Write/7  "<Buffer_7>"
  Bus Selector/8 -> Data Store Write/8  "<Buffer_8>"
  [CAN1_msg_coherent_TAG] -> Desync calculation/2(New_msg_CAN1)
  Demux message CAN1 and check coherence/3(CAN1_msg_coherent) -> [CAN1_msg_coherent_TAG], Switch/2, OR/1
  [new_msg_Rx_TAG] -> Desync calculation/Enable
  OR/1 -> [new_msg_Rx_TAG], Data Store Write2/1
  TM_COMM/1 -> Desync calculation/1(TM_COMM)
  [msg_count_CAN1] -> Desync calculation/3(msg_count_CAN1)
  [msg_count_CAN2] -> Desync calculation/4(msg_count_CAN2)

== system HANcoder_E407_TTA_Controller_v3/HANcoder STM32 Target - E407-STM32 algorithm/TTA CAN System/TTA System/Matrix Cycle Manager/Controller Matrix Cycle/controller basic cycle 1/COMP Task - Sync bc1 check/Reset Tx msg counter ==
  Enable : EnablePort
  Constant1 : Constant  Priority=2
  Constant6 : Constant  Priority=2
  Data Store Write1 : DataStoreWrite  Priority=4  DataStoreName=Tx_msg_count_CAN1
  Data Store Write2 : DataStoreWrite  Priority=4  DataStoreName=Tx_msg_count_CAN2
  wires:
  Constant6/1 -> Data Store Write1/1
  Constant1/1 -> Data Store Write2/1

== system HANcoder_E407_TTA_Controller_v3/HANcoder STM32 Target - E407-STM32 algorithm/TTA CAN System/TTA System/Matrix Cycle Manager/Controller Matrix Cycle/controller basic cycle 1/COMP Task - TMR/TMR_load_msgs_1 ==
  note: STEP 1 - Gather Output1 and Output2 messages
  note: Logic Analyzer - DEBUG
      | LT Update COMP task
      | activation
  note: Logic Analyzer - DEBUG
  Enable : EnablePort
  Bus Selector : BusSelector  OutputSignals=Buffer_2,Buffer_3,Buffer_4,Buffer_5,Buffer_6,Buffer_7
  Constant{9..12} (4 alike) : Constant  Value=torque_precision
  Constant8 : Constant  Priority=28  OutDataTypeStr=boolean
  Data Store Read : DataStoreRead  DataStoreName=output_control1_msg
  Data Store Write : DataStoreWrite  Priority=1  DataStoreName=tau_fr_out1
  Data Store Write1 : DataStoreWrite  Priority=2  DataStoreName=tau_fl_out1
  Data Store Write19 : DataStoreWrite  Priority=29  DataStoreName=Toggle_Pin_A0
  Data Store Write2 : DataStoreWrite  Priority=3  DataStoreName=tau_ar_out1
  Data Store Write3 : DataStoreWrite  Priority=4  DataStoreName=tau_al_out1
  Data Store Write4 : DataStoreWrite  Priority=5  DataStoreName=set_miss_out1
  Data Store Write5 : DataStoreWrite  Priority=6  DataStoreName=sensor_miss_out1
  uint8_2float : Subsystem
  uint8_2float1 : Subsystem
  uint8_2float2 : Subsystem
  uint8_2float3 : Subsystem
  wires:
  Data Store Read/1 -> Bus Selector/1
  Bus Selector/1 -> uint8_2float/2(value)  "<Buffer_2>"
  Bus Selector/2 -> uint8_2float1/2(value)  "<Buffer_3>"
  Bus Selector/3 -> uint8_2float2/2(value)  "<Buffer_4>"
  Bus Selector/4 -> uint8_2float3/2(value)  "<Buffer_5>"
  Bus Selector/5 -> Data Store Write4/1  "<Buffer_6>"
  Bus Selector/6 -> Data Store Write5/1  "<Buffer_7>"
  Constant8/1 -> Data Store Write19/1
  Constant9/1 -> uint8_2float/1(precision)
  uint8_2float/1(decoded) -> Data Store Write/1  "torque_fr_out1_s"
  Constant10/1 -> uint8_2float1/1(precision)
  Constant11/1 -> uint8_2float2/1(precision)
  Constant12/1 -> uint8_2float3/1(precision)
  uint8_2float1/1(decoded) -> Data Store Write1/1  "torque_fl_out1_s"
  uint8_2float2/1(decoded) -> Data Store Write2/1  "torque_ar_out1_s"
  uint8_2float3/1(decoded) -> Data Store Write3/1  "torque_al_out1_s"

== system HANcoder_E407_TTA_Controller_v3/HANcoder STM32 Target - E407-STM32 algorithm/TTA CAN System/TTA System/Matrix Cycle Manager/Controller Matrix Cycle/controller basic cycle 1/COMP Task - TMR/TMR_load_msgs_2 ==
  note: Logic Analyzer - DEBUG
  note: Logic Analyzer - DEBUG
      | LT Update COMP task
      | activation
  note: STEP 1 - Gather Output1 and Output2 messages
  Enable : EnablePort
  Bus Selector1 : BusSelector  OutputSignals=Buffer_2,Buffer_3,Buffer_4,Buffer_5,Buffer_6,Buffer_7
  Constant{13..16} (4 alike) : Constant  Value=torque_precision
  Constant8 : Constant  Priority=28  OutDataTypeStr=boolean
  Data Store Read1 : DataStoreRead  DataStoreName=output_control2_msg
  Data Store Write10 : DataStoreWrite  Priority=11  DataStoreName=set_miss_out2
  Data Store Write11 : DataStoreWrite  Priority=12  DataStoreName=sensor_miss_out2
  Data Store Write19 : DataStoreWrite  Priority=29  DataStoreName=Toggle_Pin_A0
  Data Store Write6 : DataStoreWrite  Priority=7  DataStoreName=tau_fr_out2
  Data Store Write7 : DataStoreWrite  Priority=8  DataStoreName=tau_fl_out2
  Data Store Write8 : DataStoreWrite  Priority=9  DataStoreName=tau_ar_out2
  Data Store Write9 : DataStoreWrite  Priority=10  DataStoreName=tau_al_out2
  uint8_2float4 : Subsystem
  uint8_2float5 : Subsystem
  uint8_2float6 : Subsystem
  uint8_2float7 : Subsystem
  wires:
  uint8_2float4/1(decoded) -> Data Store Write6/1  "torque_fr_out2_s"
  uint8_2float5/1(decoded) -> Data Store Write7/1  "torque_fl_out2_s"
  uint8_2float6/1(decoded) -> Data Store Write8/1  "torque_ar_out2_s"
  uint8_2float7/1(decoded) -> Data Store Write9/1  "torque_al_out2_s"
  Constant16/1 -> uint8_2float7/1(precision)
  Constant15/1 -> uint8_2float6/1(precision)
  Constant14/1 -> uint8_2float5/1(precision)
  Bus Selector1/1 -> uint8_2float4/2(value)  "<Buffer_2>"
  Constant13/1 -> uint8_2float4/1(precision)
  Constant8/1 -> Data Store Write19/1
  Data Store Read1/1 -> Bus Selector1/1
  Bus Selector1/2 -> uint8_2float5/2(value)  "<Buffer_3>"
  Bus Selector1/3 -> uint8_2float6/2(value)  "<Buffer_4>"
  Bus Selector1/4 -> uint8_2float7/2(value)  "<Buffer_5>"
  Bus Selector1/5 -> Data Store Write10/1  "<Buffer_6>"
  Bus Selector1/6 -> Data Store Write11/1  "<Buffer_7>"
